simulink model "ParameterEstimationForLine"  (R2019b)
settings: Solver=VariableStepAuto  StartTime=0.0  StopTime=10.0  RelTol=1e-3
undefined symbols (not defined in the file): b, k
settings Model: OrderedModelArguments=off  Creator=nikit  LastModifiedBy=nikit

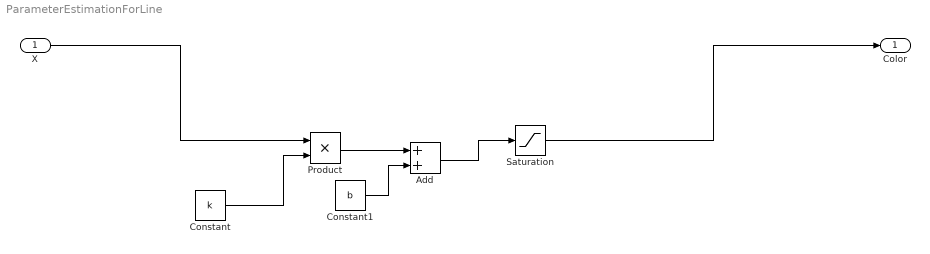
== system ParameterEstimationForLine ==
  X : Inport
  Add : Sum
  Constant : Constant  Value=k
  Constant1 : Constant  Value=b
  Product : Product
  Saturation : Saturate  UpperLimit=32  LowerLimit=3
  Color : Outport
  wires:
  Saturation/1 -> Color/1
  X/1 -> Product/1
  Product/1 -> Add/1
  Add/1 -> Saturation/1
  Constant/1 -> Product/2
  Constant1/1 -> Add/2
